simulink model "interpolation_nD_TestGen19"  (R2017b)
settings: Solver=FixedStepDiscrete  StartTime=0.0  StopTime=10.0  RelTol=1e-3
settings Model: Creator=ktrinh  LastModifiedBy=ktrinh
settings DebuggingCC: ParameterOverflowMsg=none

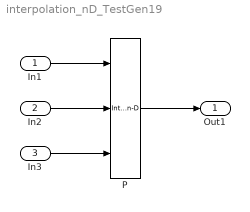
== system interpolation_nD_TestGen19 ==
  In1 : Inport  OutMin=0  OutMax=2  PortDimensions=3
  In2 : Inport  Port=2  OutMin=-0.5  OutMax=1.5
  In3 : Inport  Port=3  OutMin=0  OutMax=5
  P : Interpolation_n-D  Table=[24.2644332556736 40.1142002355637 55.7886663041661 6.24538107172769 75.1114661193454;116.07629477507 13.809417058981 68.3102874359306 70.0321877271685 34.9558503864397]  InterpMethod=Flat  ExtrapMethod=Clip  ValidIndexMayReachLast=on  NumSelectionDims=1  OutDataTypeStr=uint32  InternalRulePriority=Speed  RndMeth=Simplest  SaturateOnIntegerOverflow=on
      settings: InputPortMap=u0,u1,u2
  Out1 : Outport
  wires:
  In1/1 -> P/1
  In2/1 -> P/2
  In3/1 -> P/3
  P/1 -> Out1/1
